simulink model "add"  (R2022b)
settings: Solver=VariableStepAuto  StartTime=0.0  StopTime=inf  RelTol=1e-3
InitFcn:
  | x=176;
  | y=2;
  | k=2;
StartFcn:
  | x=10;
PostSaveFcn:
  | x=176;
  | y=2;
  | k=2;
CloseFcn:
  | clear x;
  | clear y;
  | clear k;
PauseFcn:
  | x=1;
ContinueFcn:
  | x=198;
settings Model: Creator=Brigosha_Guest  LastModifiedBy=Brigosha_Guest

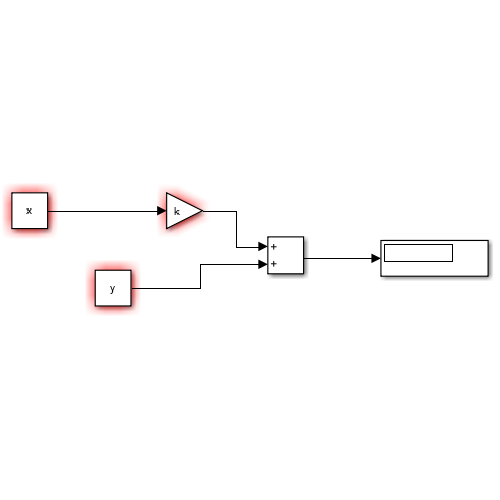
[thumbnail: Simulink's stored preview of the top-level diagram]
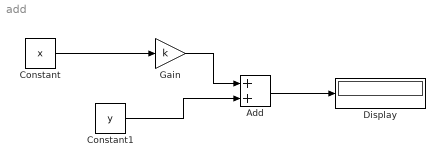
== system add ==
  Add : Sum
  Constant : Constant  Value=x
  Constant1 : Constant  Value=y
  Display : Display
  Gain : Gain  Gain=k
  wires:
  Constant/1 -> Gain/1
  Gain/1 -> Add/1
  Constant1/1 -> Add/2
  Add/1 -> Display/1
